simulink model "hdlcoderdft"  (R2017a)
settings: Solver=FixedStepDiscrete  StartTime=0.0  StopTime=10.0  RelTol=1e-3
InitFcn:
  | hdlcoderdft_init
values from neighbouring files (symbols this model uses):
  nDistances = 4    [hdlcoderdft_init.m]
  nFilters = 4    [hdlcoderdft_init.m]
settings Model: DataTypeOverride=Off  Creator=Pierre BERNARDI  LastModifiedBy=Pierre BERNARDI
settings DataIOCC: LimitDataPoints=on  SaveOutput=off  SaveTime=off
settings OptimizationCC: BlockReduction=off  ConditionallyExecuteInputs=off  DefaultParameterBehavior=Inlined  LifeSpan=inf
settings DebuggingCC: AlgebraicLoopMsg=error  SingleTaskRateTransMsg=error  AllowSymbolicDim=off  StrictBusMsg=ErrorOnBusTreatedAsVector  SFUnexpectedBacktrackingDiag=warning  SFNoUnconditionalDefaultTransitionDiag=warning  SFExecutionAtInitializationDiag=none
settings HardwareCC: ProdBitPerPointer=32  ProdBitPerSizeT=32  ProdBitPerPtrDiffT=32  ProdLargestAtomicFloat=None  ProdIntDivRoundTo=Undefined  ProdEndianess=Unspecified  ProdWordSize=32  ProdHWDeviceType=ASIC/FPGA->ASIC/FPGA  ProdEqTarget=off
settings GRTTargetCC: TargetLangStandard=C89/C90 (ANSI)  GeneratePreprocessorConditionals=Disable all
settings ConfigComp: CovScope=ReferencedModels  CovMetricSettings=dw  CovHtmlReporting=on  CovSaveCumulativeToWorkspaceVar=on  CovSaveSingleToWorkspaceVar=on  CovExternalEMLEnable=off  CovSFcnEnable=off

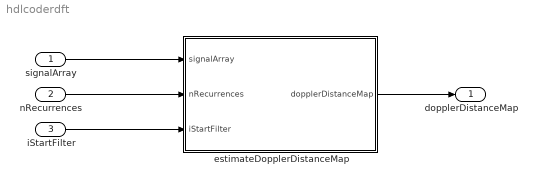
== system hdlcoderdft ==
  signalArray : Inport  OutDataTypeStr=double  PortDimensions=[1 800*51]  Interpolate=off
      settings: VarSizeSig=Yes  SignalType=complex
  nRecurrences : Inport  Port=2  OutMin=125  OutMax=800  OutDataTypeStr=uint16
  iStartFilter : Inport  Port=3  OutDataTypeStr=uint16
  estimateDopplerDistanceMap : MATLAB Function  TreatAsAtomicUnit=on
  dopplerDistanceMap : Outport  OutDataTypeStr=double
      settings: SignalType=complex
  wires:
  signalArray/1 -> estimateDopplerDistanceMap/1(signalArray)
  nRecurrences/1 -> estimateDopplerDistanceMap/2(nRecurrences)
  iStartFilter/1 -> estimateDopplerDistanceMap/3(iStartFilter)
  estimateDopplerDistanceMap/1(dopplerDistanceMap) -> dopplerDistanceMap/1

== matlab function hdlcoderdft/estimateDopplerDistanceMap ==
  data: signalArray input size=[1 800*51]; dopplerDistanceMap output; nRecurrences input [125..800]; iStartFilter input; nDistances parameter; nFilters parameter
function dopplerDistanceMap = estimateDopplerDistanceMap(signalArray, nRecurrences, iStartFilter, nDistances, nFilters)
    nSamplesMax = 51 * 800
    coder.varsize('signalArray', [1 nSamplesMax])
    dopplerDistanceMap = zeros(nDistances, nFilters)
